simulink model "EditingJohnsInitiateAndZeroFunctions"  (R2021a)
settings: Solver=VariableStepAuto  StartTime=0.0  StopTime=10.0  RelTol=1e-3
model workspace (MAT data in the model file):
  ID = 1
undefined symbols (not defined in the file or in its folder): A, C, SendOnlyCommand
libraries: speedgoatlib_IO691 x4, canmsglib x2, slrealtimeutilitieslib x1
settings Model: Creator=kylec  LastModifiedBy=kylec

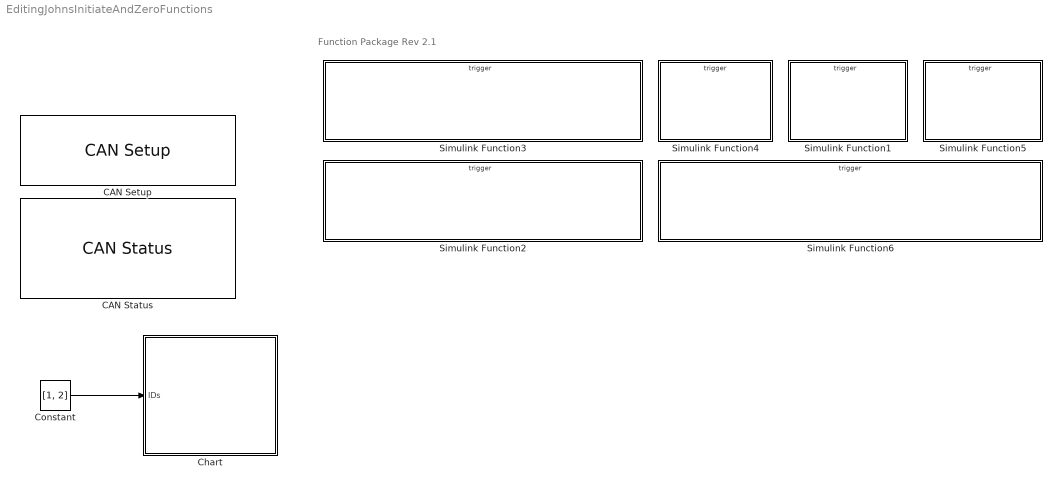
== system EditingJohnsInitiateAndZeroFunctions ==
  note: Function Package Rev 2.1
  "CAN Setup " : speedgoatlib_IO691/CAN Setup   moduletype=IO691  id=1  pciSlot=-1  chn1=CAN (HS)  chn2=CAN (HS)  chn3=Disabled  chn4=Disabled  initStruct=[]  termStruct=[]  ArbitrationbdrChn1=1.0 MBaud  ArbitrationManbdrChn1=[2,8,31,8]  FdbdrChn1=5.0 MBaud  FdManbdrChn1=[2,2,5,2]  ArbitrationbdrChn2=1.0 MBaud  ArbitrationManbdrChn2=[2,8,31,8]  FdbdrChn2=5.0 MBaud  FdManbdrChn2=[2,2,5,2]  ArbitrationbdrChn3=1.0 MBaud  ArbitrationManbdrChn3=[2,8,31,8]  FdbdrChn3=5.0 MBaud  FdManbdrChn3=[2,2,5,2]  ArbitrationbdrChn4=1.0 MBaud  ArbitrationManbdrChn4=[2,8,31,8]  FdbdrChn4=5.0 MBaud  FdManbdrChn4=[2,2,5,2]  moduleInitValues=[691 1 -1 -1]
      settings: SourceProductName=Simulink Real-Time: Speedgoat I/O Blockset
  CAN Status : speedgoatlib_IO691/CAN Status  moduleId=1  sampleTime=-1  channel=1  busRecovery=Off  arrayOutput=off  controllerCpuLoad=off  controllerLiveCount=off  initModeAct=off  avgBusLoad=off  receiving=off  RxQueueEmpty=off  dataOverrunRcv=off  rxBufferLevel=off  txPending=off  dataOverrunTx=off  txBufferLevel=off  errWarnLimit=off  errPassLimit=off  errBusOff=off  busRecoveryCounter=off  busCouplingErr=off  transceiverErr=off  opMode=off  brp=off  timeSegment1=off  timeSegment2=off  synchronisationJumpWidth=off  dataTSEG1=off  dataTSEG2=off  dataSJW=off  moduleType=691  qtyStatBlk=1  ptIdx=0  isFDMod=0
      settings: SourceProductName=Simulink Real-Time: Speedgoat I/O Blockset
  Chart : Stateflow chart  TreatAsAtomicUnit=on
  Constant : Constant  Value=[1, 2]
  Simulink Function1 : Subsystem  TreatAsAtomicUnit=on
  Simulink Function2 : Subsystem  TreatAsAtomicUnit=on
  Simulink Function3 : Subsystem  TreatAsAtomicUnit=on
  Simulink Function4 : Subsystem  TreatAsAtomicUnit=on
  Simulink Function5 : Subsystem  TreatAsAtomicUnit=on
  Simulink Function6 : Subsystem  TreatAsAtomicUnit=on
  wires:
  Constant/1 -> Chart/1(IDs)

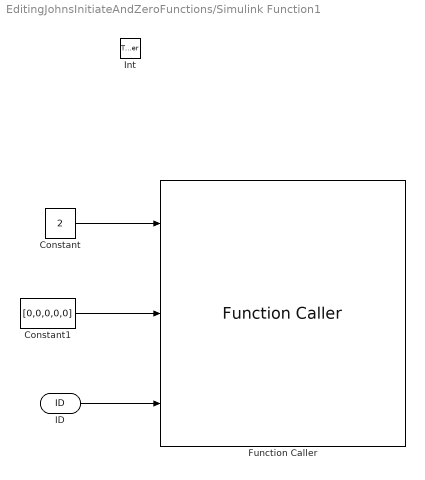
== system EditingJohnsInitiateAndZeroFunctions/Simulink Function1 ==
  Int : TriggerPort  TriggerType=function-call  IsSimulinkFunction=on  FunctionName=Int  FunctionVisibility=scoped  VariantControl=(inherit)
  Constant : Constant  Value=2
  Constant1 : Constant  Value=[0,0,0,0,0]
  Function Caller : FunctionCaller  FunctionPrototype=SendOnlyCommand(C,A,ID)  InputArgumentSpecifications=<Enter example>  OutputArgumentSpecifications=<Enter example>
  ID : ArgIn  ArgumentName=ID
  wires:
  ID/1 -> Function Caller/3
  Constant1/1 -> Function Caller/2
  Constant/1 -> Function Caller/1

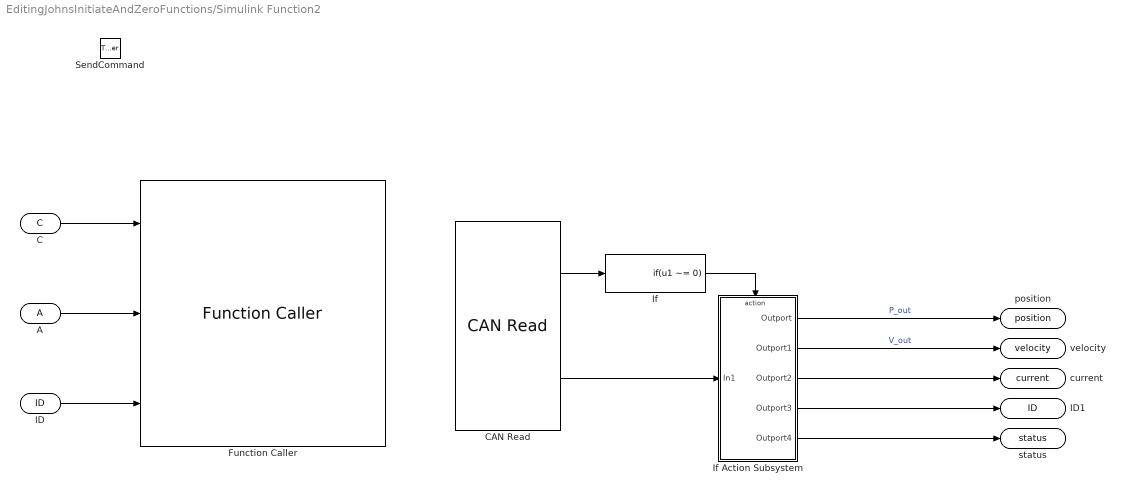
== system EditingJohnsInitiateAndZeroFunctions/Simulink Function2 ==
  SendCommand : TriggerPort  TriggerType=function-call  IsSimulinkFunction=on  FunctionName=SendCommand  FunctionVisibility=scoped  VariantControl=(inherit)
  CAN Read : speedgoatlib_IO691/CAN Read  id=1  ts=-1  channel=1  messageType=CAN  canType=CAN (HS)  initValues=[691 1 -1 0 1 1]
      settings: SourceProductName=Simulink Real-Time: Speedgoat I/O Blockset
  Function Caller : FunctionCaller  FunctionPrototype=SendOnlyCommand(C,A,ID)  InputArgumentSpecifications=<Enter example>  OutputArgumentSpecifications=<Enter example>
  If : If  IfExpression=u1 ~= 0  ShowElse=off
  If Action Subsystem : Subsystem  TreatAsAtomicUnit=on
  C : ArgIn  DisableCoverage=on  ArgumentName=C
  A : ArgIn  Port=2  PortDimensions=5  ArgumentName=A
  ID : ArgIn  Port=3  ArgumentName=ID
  position : ArgOut  ArgumentName=position
  velocity : ArgOut  Port=2  ArgumentName=velocity
  current : ArgOut  Port=3  ArgumentName=current
  ID1 : ArgOut  Port=4  ArgumentName=ID
  status : ArgOut  Port=5  OutDataTypeStr=uint8  ArgumentName=status
  wires:
  CAN Read/1 -> If/1
  If/1 -> If Action Subsystem/Action
  If Action Subsystem/3(Outport2) -> current/1
  If Action Subsystem/4(Outport3) -> ID1/1
  If Action Subsystem/5(Outport4) -> status/1
  If Action Subsystem/2(Outport1) -> velocity/1  "V_out"
  CAN Read/2 -> If Action Subsystem/1(In1)
  If Action Subsystem/1(Outport) -> position/1  "P_out"
  C/1 -> Function Caller/1
  ID/1 -> Function Caller/3
  A/1 -> Function Caller/2

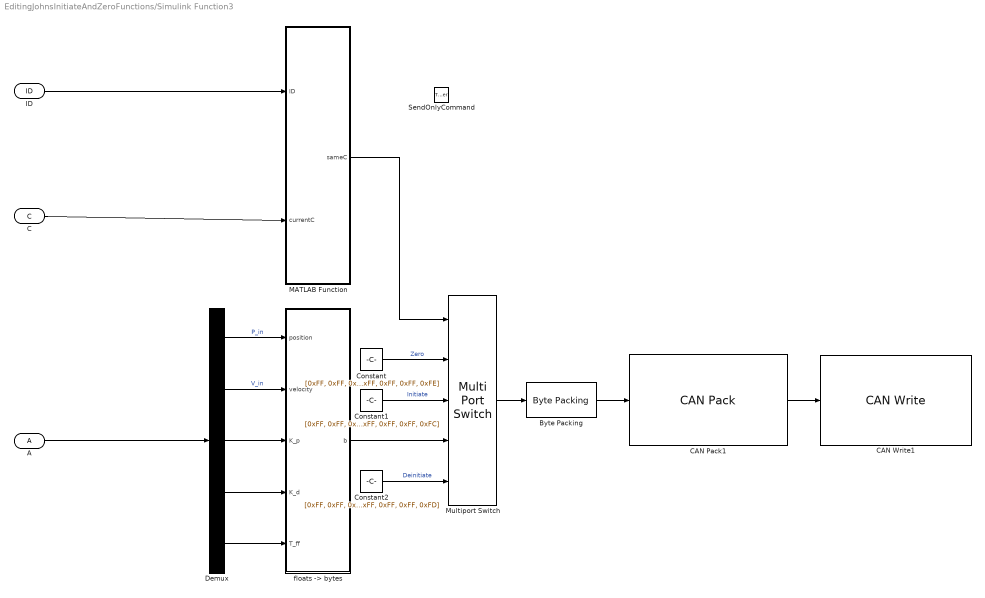
== system EditingJohnsInitiateAndZeroFunctions/Simulink Function3 ==
  SendOnlyCommand : TriggerPort  TriggerType=function-call  IsSimulinkFunction=on  FunctionName=SendOnlyCommand  FunctionVisibility=scoped  VariantControl=(inherit)
  Byte Packing : slrealtimeutilitieslib/Byte Packing  MaskPackedDataType=uint8  MaskUnpackedDataTypes={['uint8']}  MaskAlignment=1
  CAN Pack1 : canmsglib/CAN Pack  MsgList=(none)  MsgName=CAN Msg  MsgIDType=Standard (11-bit identifier)  MsgIdentifier=ID  MsgLength=8  Remote=off  ApplyMinMax=off  BusOutput=off  SignalInfo={ 'b1', '0', '8', 'LE', 'unsigned', 'Standard', '0', '1', '0', '-Inf', 'Inf'; 'b2', '8', '8', 'LE', 'unsigned', 'Standard', '0', '1', '0', '-Inf', 'Inf'; 'b3', '16', '8', 'LE', 'unsigned', 'Standard', '0', '1', '0', '-Inf', 'Inf'; 'b4', '24', '8', 'LE', 'unsigned', 'Standard', '0', '1', '0', '-Inf', 'Inf'; 'b5', '32', '8', 'LE', 'unsigned', 'Standard', '0', '1', '0', '-Inf', 'Inf'; 'b6', '40', '8', 'LE', 'unsigned', 'Standard', '0', '1', '0', '-Inf', 'Inf'; 'b7', '48', '8', 'LE', 'unsigned', 'Standard', '0', '1', '0', '-Inf', 'Inf'; 'b8', '56', '8', 'LE', 'unsigned', 'Standard', '0', '1', '0', '-Inf', 'Inf' }
      settings: SourceProductBaseCode=ME,XP,VN  DataFormat=raw data
  CAN Write1 : speedgoatlib_IO691/CAN Write  id=1  ts=-1  channel=1  messageType=CAN  enableStatusPort=off  canType=CAN (HS)  initValues=[691 1 -1 0 1 1 0]
      settings: SourceProductName=Simulink Real-Time: Speedgoat I/O Blockset
  Constant : Constant  Value=[0xFF, 0xFF, 0xFF, 0xFF, 0xFF, 0xFF, 0xFF, 0xFE]
  Constant1 : Constant  Value=[0xFF, 0xFF, 0xFF, 0xFF, 0xFF, 0xFF, 0xFF, 0xFC]
  Constant2 : Constant  Value=[0xFF, 0xFF, 0xFF, 0xFF, 0xFF, 0xFF, 0xFF, 0xFD]
  Demux : Demux  Outputs=5
  MATLAB Function : MATLAB Function  TreatAsAtomicUnit=on
  Multiport Switch : MultiPortSwitch  Inputs=4
  "floats -> bytes" : MATLAB Function  TreatAsAtomicUnit=on
  C : ArgIn  DisableCoverage=on  ArgumentName=C
  A : ArgIn  Port=2  PortDimensions=5  ArgumentName=A
  ID : ArgIn  Port=3  ArgumentName=ID
  wires:
  Demux/5 -> "floats -> bytes"/5(T_ff)
  Multiport Switch/1 -> Byte Packing/1
  Demux/4 -> "floats -> bytes"/4(K_d)
  Demux/1 -> "floats -> bytes"/1(position)  "P_in"
  Constant/1 -> Multiport Switch/2  "Zero"
  Demux/2 -> "floats -> bytes"/2(velocity)  "V_in"
  Constant2/1 -> Multiport Switch/5  "Deinitiate"
  CAN Pack1/1 -> CAN Write1/1
  Byte Packing/1 -> CAN Pack1/1
  Constant1/1 -> Multiport Switch/3  "Initiate"
  "floats -> bytes"/1(b) -> Multiport Switch/4
  Demux/3 -> "floats -> bytes"/3(K_p)
  MATLAB Function/1(sameC) -> Multiport Switch/1
  C/1 -> MATLAB Function/2(currentC)
  ID/1 -> MATLAB Function/1(ID)
  A/1 -> Demux/1

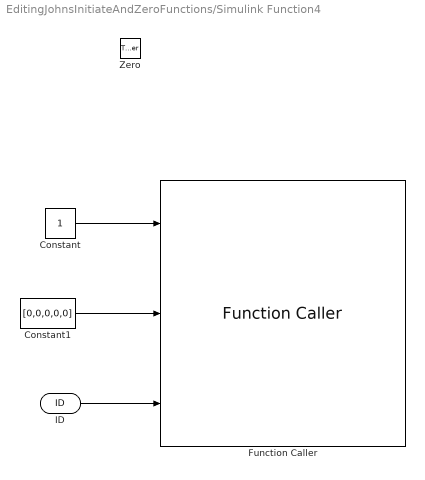
== system EditingJohnsInitiateAndZeroFunctions/Simulink Function4 ==
  Zero : TriggerPort  TriggerType=function-call  IsSimulinkFunction=on  FunctionName=Zero  FunctionVisibility=scoped  VariantControl=(inherit)
  Constant : Constant
  Constant1 : Constant  Value=[0,0,0,0,0]
  Function Caller : FunctionCaller  FunctionPrototype=SendOnlyCommand(C,A,ID)  InputArgumentSpecifications=<Enter example>  OutputArgumentSpecifications=<Enter example>
  ID : ArgIn  ArgumentName=ID
  wires:
  ID/1 -> Function Caller/3
  Constant1/1 -> Function Caller/2
  Constant/1 -> Function Caller/1

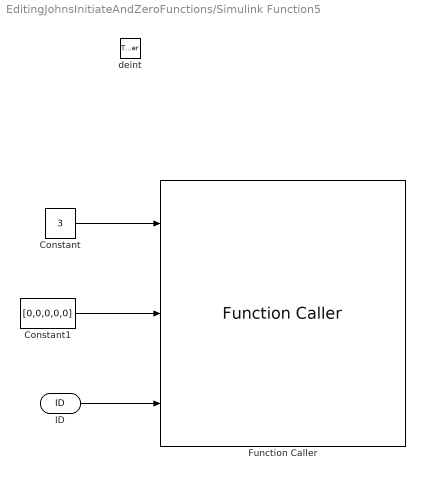
== system EditingJohnsInitiateAndZeroFunctions/Simulink Function5 ==
  deint : TriggerPort  TriggerType=function-call  IsSimulinkFunction=on  FunctionName=deint  FunctionVisibility=scoped  VariantControl=(inherit)
  Constant : Constant  Value=3
  Constant1 : Constant  Value=[0,0,0,0,0]
  Function Caller : FunctionCaller  FunctionPrototype=SendOnlyCommand(C,A,ID)  InputArgumentSpecifications=<Enter example>  OutputArgumentSpecifications=<Enter example>
  ID : ArgIn  ArgumentName=ID
  wires:
  ID/1 -> Function Caller/3
  Constant1/1 -> Function Caller/2
  Constant/1 -> Function Caller/1

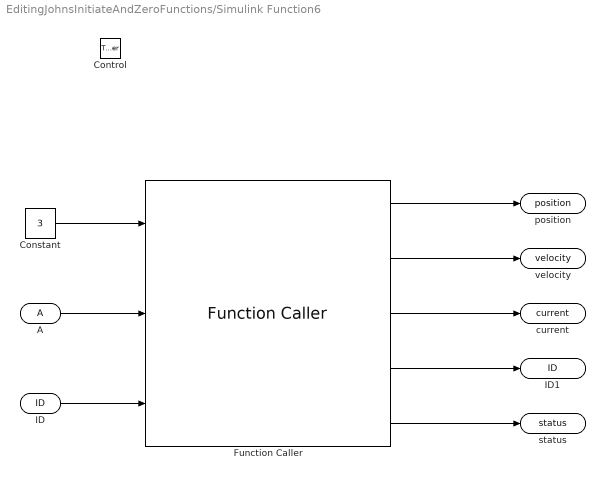
== system EditingJohnsInitiateAndZeroFunctions/Simulink Function6 ==
  Control : TriggerPort  TriggerType=function-call  IsSimulinkFunction=on  FunctionName=Control  FunctionVisibility=scoped  VariantControl=(inherit)
  Constant : Constant  Value=3
  Function Caller : FunctionCaller  FunctionPrototype=[position,velocity,current,ID,status] = SendCommand(C,A,ID)  InputArgumentSpecifications=<Enter example>  OutputArgumentSpecifications=<Enter example>
  A : ArgIn  PortDimensions=5  ArgumentName=A
  ID : ArgIn  Port=2  ArgumentName=ID
  position : ArgOut  ArgumentName=position
  velocity : ArgOut  Port=2  ArgumentName=velocity
  current : ArgOut  Port=3  ArgumentName=current
  ID1 : ArgOut  Port=4  ArgumentName=ID
  status : ArgOut  Port=5  OutDataTypeStr=uint8  ArgumentName=status
  wires:
  Constant/1 -> Function Caller/1
  A/1 -> Function Caller/2
  ID/1 -> Function Caller/3
  Function Caller/4 -> ID1/1
  Function Caller/1 -> position/1
  Function Caller/2 -> velocity/1
  Function Caller/3 -> current/1
  Function Caller/5 -> status/1

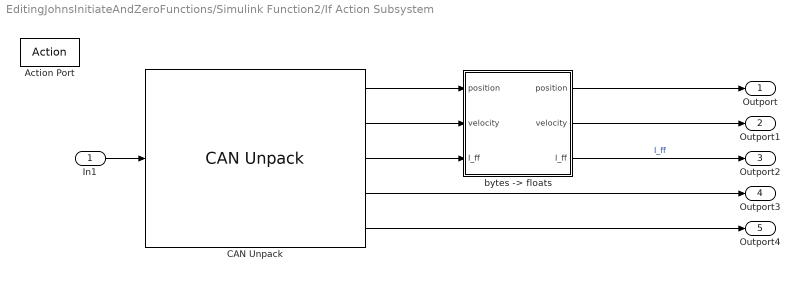
== system EditingJohnsInitiateAndZeroFunctions/Simulink Function2/If Action Subsystem ==
  In1 : Inport
  Action Port : ActionPort  ActionPortLabel=if(u1 ~= 0)
  CAN Unpack : canmsglib/CAN Unpack  MsgList=(none)  MsgName=CAN Msg  MsgIDType=Standard (11-bit identifier)  MsgIdentifier=-1  MsgLength=6  SignalInfo={ 'position', '16', '16', 'BE', 'unsigned', 'Standard', '0', '1', '0', '0', '65535'; 'velocity', '36', '12', 'BE', 'unsigned', 'Standard', '0', '1', '0', '0', '4095'; 'current', '40', '12', 'BE', 'unsigned', 'Standard', '0', '1', '0', '0', '4095'; 'id', '0', '8', 'BE', 'unsigned', 'Standard', '0', '1', '0', '0', '255' }  IDPort=off  TimestampPort=off  ErrorPort=off  RemotePort=off  LengthPort=off  StatusPort=on  ApplyMinMax=off
      settings: SourceProductBaseCode=ME,XP,VN
  "bytes -> floats" : MATLAB Function  TreatAsAtomicUnit=on
  Outport : Outport
  Outport1 : Outport  Port=2
  Outport2 : Outport  Port=3
  Outport3 : Outport  Port=4
  Outport4 : Outport  Port=5
  wires:
  CAN Unpack/5 -> Outport4/1
  CAN Unpack/1 -> "bytes -> floats"/1("position ")
  CAN Unpack/3 -> "bytes -> floats"/3("I_ff ")
  "bytes -> floats"/1(position) -> Outport/1
  CAN Unpack/4 -> Outport3/1
  "bytes -> floats"/2(velocity) -> Outport1/1
  "bytes -> floats"/3(I_ff) -> Outport2/1  "I_ff"
  CAN Unpack/2 -> "bytes -> floats"/2("velocity ")
  In1/1 -> CAN Unpack/1

== matlab function EditingJohnsInitiateAndZeroFunctions/Simulink Function2/If Action Subsystem/bytes -> floats ==
  data: position input; position output; velocity output; I_ff output; velocity input; I_ff input
function [position, velocity, I_ff] = fcn(position, velocity, I_ff)

P_MIN  =-95.5;  % [rad]
P_MAX  = 95.5;  % [rad]
V_MIN  =-45;    % [rad/s]
V_MAX  = 45;    % [rad/s]
I_MIN  =-40;    % []
I_MAX  = 40;    % []

position = position*(P_MAX  - P_MIN)/65535+ P_MIN;
velocity = velocity*(V_MAX  - V_MIN)/4095 + V_MIN;
I_ff     = I_ff*(I_MAX  - I_MIN)/4095 + I_MIN;

== stateflow chart EditingJohnsInitiateAndZeroFunctions/Chart ==
  state Zero
    (default) -> (junction 119) : % currID
    (junction 119) -> (junction 121) : {i = 1;}
    (junction 121) -> (junction 120) [order 1] : [i < length(IDs) + 1]
    (junction 120) -> (junction 122) : {currID = IDs(i);
        | Zero(currID);}
    (junction 123) -> (junction 121)
    (junction 121) -> (junction 124) [order 2]
    (junction 122) -> (junction 123) : {i = i + 1;}
  state Cycle [commented out]
    entry:
    Int(ID);
  state step [commented out]
    ID = ID +1
  state Initiate
    (default) -> (junction 155) : % currID
        | {currID = 0}
    (junction 155) -> (junction 157) : {i = 1;}
    (junction 157) -> (junction 150) [order 1] : [i < length(IDs)]
    (junction 150) -> (junction 158) : {currID = IDs(i);
        | Int(currID);}
    (junction 156) -> (junction 157)
    (junction 157) -> (junction 159) [order 2]
    (junction 158) -> (junction 156) : {i = i + 1;}
  (default) -> Zero
  step -> Cycle [commented out] : [after(.1,sec)]
  Cycle -> step [commented out] : [(ID < MaxID)]
  Zero -> Initiate
  data: IDs input; i local double; currID local

== matlab function EditingJohnsInitiateAndZeroFunctions/Simulink Function3/floats -> bytes ==
  data: position input; b output uint8 size=8; velocity input; K_p input; K_d input; T_ff input
function b = fcn(position, velocity, K_p, K_d, T_ff)

P_MIN  =-95.5;  % [rad]
P_MAX  = 95.5;  % [rad]
V_MIN  =-45;    % [rad/s] 30 to 45
V_MAX  = 45;    % [rad/s]
KP_MIN = 0;     % [Nm/rad]
KP_MAX = 500;   % [Nm/rad]
KD_MIN = 0;     % [Nm*s/rad
KD_MAX = 5;     % [Nm*s/rad
T_MIN  =-18;    % [Nm]
T_MAX  = 18;    % [Nm]

position = floor((max(min(position,P_MAX) ,P_MIN)  - P_MIN )*65535/(P_MAX  - P_MIN));
velocity = floor((max(min(velocity,V_MAX) ,V_MIN)  - V_MIN )*4095 /(V_MAX  - V_MIN));
K_p      = floor((max(min(K_p     ,KP_MAX),KP_MIN) - KP_MIN)*4095 /(KP_MAX - KP_MIN));
K_d      = floor((max(min(K_d     ,V_MAX) ,V_MIN)  - KD_MIN)*4095 /(KD_MAX - KD_MIN));
T_ff     = floor((max(min(T_ff    ,V_MAX) ,V_MIN)  - T_MIN )*4095 /(T_MAX  - T_MIN));

p  = dec2bin(position);
p  = [repmat('0', 1, 16-length(p)),p];
v  = dec2bin(velocity);
v  = [repmat('0', 1, 12-length(v)),v];
kp = dec2bin(K_p);
kp  = [repmat('0', 1, 12-length(kp)),kp];
kd = dec2bin(K_d);
kd  = [repmat('0', 1, 12-length(kd)),kd];
t  = dec2bin(T_ff);
t  = [repmat('0', 1, 12-length(t)),t];

B = repmat('0', 8, 8);

B(1,:) = p(1:8);
B(2,:) = p(9:16);
B(3,:) = v(1:8);
B(4,:) = [v(9:12),kp(1:4)];
B(5,:) = kp(5:12);
B(6,:) = kd(1:8);
B(7,:) = [kd(9:12),t(1:4)];
B(8,:) = t(5:12);

B  = bin2dec(B);

b = uint8(B);

== matlab function EditingJohnsInitiateAndZeroFunctions/Simulink Function3/MATLAB Function ==
  data: ID input; sameC output; currentC input
function sameC = setCurrentID(ID, currentC)
% coder.extrinsic('get_param')
coder.extrinsic('assignin')
% 
% model = get_param(bdroot, 'Name');
% mws = get_param(model, 'modelworkspace');
assignin('base','ID', ID);
%display(ID);

sameC = currentC;
